simulink model "suspension_model"  (R2023b)
settings: Solver=VariableStepAuto  StartTime=0.0  StopTime=10.0  RelTol=1e-3
InitFcn:
  | suspension_params
undefined symbols (not defined in the file): h_0, h_bump, l1, l2, T, t_bump, v
libraries: simulink x1
settings Model: Creator=micha  LastModifiedBy=micha

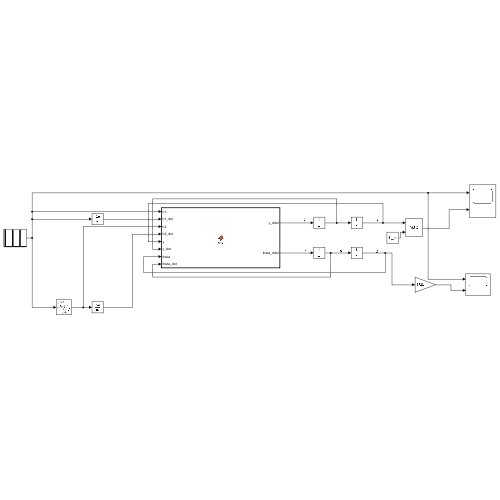
[thumbnail: Simulink's stored preview of the top-level diagram]
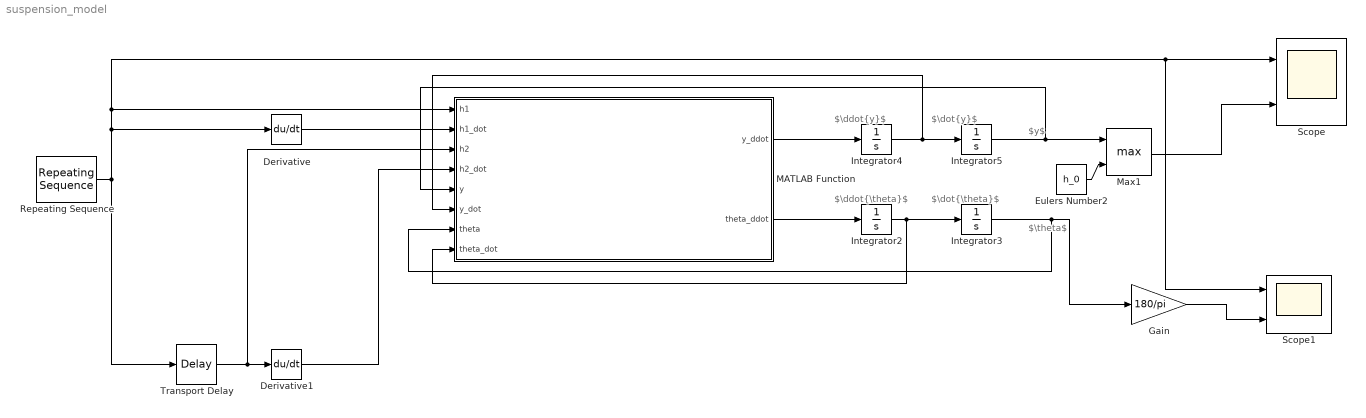
== system suspension_model ==
  note: $\ddot{\theta}$
  note: $\dot{\theta}$
  note: $\ddot{y}$
  note: $\dot{y}$
  note: $y$
  note: $\theta$
  Derivative : Derivative
  Derivative1 : Derivative
  Eulers Number2 : Constant  Value=h_0  OutDataTypeStr=Inherit: Inherit via back propagation
  Gain : Gain  Gain=180/pi
  Integrator{2..5} (4 alike) : Integrator
  MATLAB Function : MATLAB Function  TreatAsAtomicUnit=on
  Max1 : MinMax  Function=max  Inputs=2
  Repeating Sequence : simulink/Sources/Repeating Sequence  rep_seq_t="[0 2 2+t_bump*0.2  2+t_bump*0.8 2+t_bump T]"  rep_seq_y=[h_0 h_0 h_bump h_bump h_0 0]
  Scope : Scope  NumInputPorts=2
  Scope1 : Scope  NumInputPorts=2
  Transport Delay : TransportDelay  DelayTime=(l1+l2)/v
  wires:
  Repeating Sequence/1 -> Derivative/1, Scope1/1, Scope/1, MATLAB Function/1(h1), Transport Delay/1
  Integrator2/1 -> Integrator3/1, MATLAB Function/8(theta_dot)
  MATLAB Function/2(theta_ddot) -> Integrator2/1
  MATLAB Function/1(y_ddot) -> Integrator4/1
  Integrator4/1 -> MATLAB Function/6(y_dot), Integrator5/1
  Eulers Number2/1 -> Max1/2
  Integrator5/1 -> MATLAB Function/5(y), Max1/1
  Derivative/1 -> MATLAB Function/2(h1_dot)
  Transport Delay/1 -> Derivative1/1, MATLAB Function/3(h2)
  Derivative1/1 -> MATLAB Function/4(h2_dot)
  Integrator3/1 -> Gain/1, MATLAB Function/7(theta)
  Gain/1 -> Scope1/2
  Max1/1 -> Scope/2

== matlab function suspension_model/MATLAB Function ==
  data: h1 input; y_ddot output; theta_ddot output; h1_dot input; h2 input; h2_dot input; y input; y_dot input; theta input; theta_dot input
function [y_ddot, theta_ddot] = fcn(h1, h1_dot, h2, h2_dot, y, y_dot, theta, theta_dot)

g = 9.8;
m = 200;
H = 0.2;
L = 0.8;
I = 1/12 * m * (H^2 + L^2);
l1 = L/2 - L/6;
l2 = l1;
K1 = 100000;
K2 = 100000;
C1 = 400;
C2 = 400;

F1 = K1 * (h1 - (y + l1 * theta)) + C1 * (h1_dot - (y_dot + l1 * theta_dot));
F2 = K2 * (h2 - (y - l2 * theta)) + C2 * (h2_dot - (y_dot - l2 * theta_dot));
y_ddot = 1/m * (F1 + F2);
theta_ddot = 1/I * (F1 * l1 - F2 * l2);
